simulink library "lib_lqr_controller"  (R2018a)
settings: Solver=VariableStepAuto  StartTime=0.0  StopTime=10.0  RelTol=1e-3
settings Model: Creator=aj  LastModifiedBy=aj

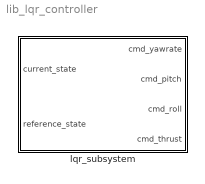
== system lib_lqr_controller ==
  lqr_subsystem : Subsystem  mask{lqr_k_matrix=[eye(3), eye(3), 0; zeros(1,6), 1], lqr_k_matrix_vel=[eye(3), eye(3), 0; zeros(1,6), 1], velcontrol_mode=off, total_mass_inair=0.85, gravity_accel=9.81}
      mask prompts: lqr_k_matrix "Feedback (fullstate) Gain Matrix [4x7]"; lqr_k_matrix_vel "Feedback (velocity) Gain Matrix [4x7]"; velcontrol_mode "Apply Only Velocity Control"; total_mass_inair "Total Flying Mass (kg)"; gravity_accel "Acceleration Due To Gravity"
      mask help:
      | This is the LQR control block.
      | Note: block color changes to 'lightBlue' if you are doing velocity-only control.
      mask Callback velcontrol_mode:
      | if( strcmp(get_param( gcb, 'velcontrol_mode' ), 'on') )
      |   set_param( gcb, 'BackgroundColor', 'lightBlue' );
      | else
      |   set_param( gcb, 'BackgroundColor', 'white' );
      | end
      mask DialogControl DescGroupVar Prompt: Nimbus LQR Block
      mask DialogControl DescTextVar Prompt: Generalized LQR feedback implemented as Simulink blocks.
      mask DialogControl Container3 Prompt: Specific Parameters

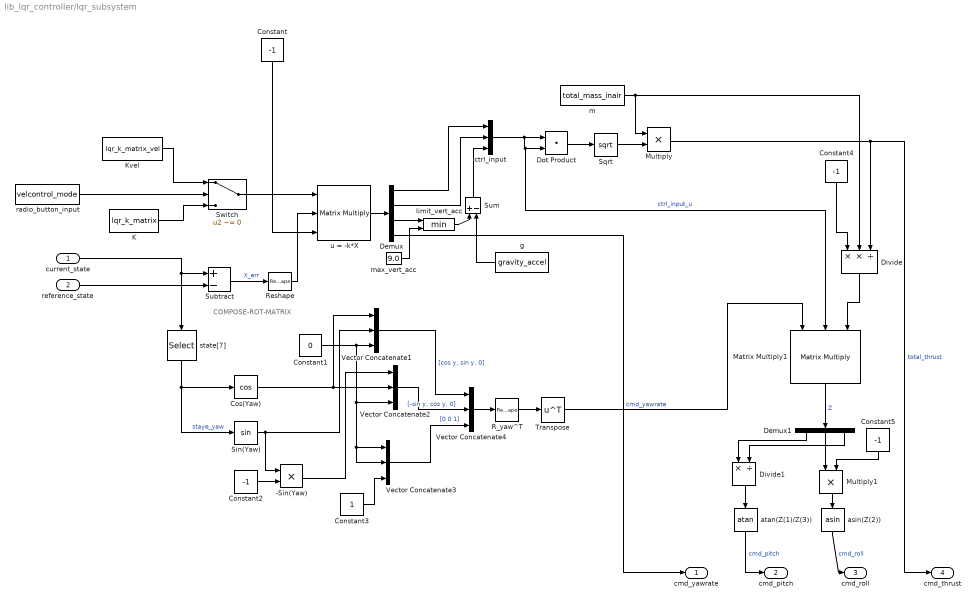
== system lib_lqr_controller/lqr_subsystem ==
  note: COMPOSE-ROT-MATRIX
  current_state : Inport  PortDimensions=7
  reference_state : Inport  Port=2
  -Sin(Yaw) : Product
  Constant{,2,4..5} (4 alike) : Constant  Value=-1
  Constant1 : Constant  Value=0
  Constant3 : Constant
  Cos(Yaw) : Trigonometry  Operator=cos
  Demux : Demux
  Demux1 : Demux  Outputs=3
  Divide : Product  Inputs=**/
  Divide1 : Product  Inputs=*/
  Dot Product : DotProduct  OutMin=0.001  InputSameDT=on  OutDataTypeStr=Inherit: Inherit via internal rule
  K : Constant  Value=lqr_k_matrix
  Kvel : Constant  Value=lqr_k_matrix_vel
  Matrix Multiply1 : Product  Inputs=3  Multiplication=Matrix(*)
  Multiply : Product
  Multiply1 : Product
  R_yaw^T : Reshape  OutputDimensionality=Customize  OutputDimensions=[3,3]
  Reshape : Reshape  OutputDimensionality=Column vector (2-D)
  Sin(Yaw) : Trigonometry
  Sqrt : Sqrt  SaturateOnIntegerOverflow=on
  Subtract : Sum  Inputs=+-
  Sum : Sum  Inputs=+-
  Switch : Switch  Criteria=u2 ~= 0
  Transpose : Math  Operator=transpose  SaturateOnIntegerOverflow=on
  Vector Concatenate{1..4} (4 alike) : Concatenate  NumInputs=3
  asin(Z(2)) : Trigonometry  Operator=asin
  atan(Z(1)/Z(3)) : Trigonometry  Operator=atan
  ctrl_input : Concatenate  NumInputs=3
  g : Constant  Value=gravity_accel
  limit_vert_acc : MinMax  Inputs=2
  m : Constant  Value=total_mass_inair
  max_vert_acc : Constant  Value=9.0
  radio_button_input : Constant  Value=velcontrol_mode
  state[7] : Selector  InputPortWidth=7  IndexOptions=Index vector (dialog)  Indices=7  OutputSizes=1
  u = -k*X : Product  Inputs=3  Multiplication=Matrix(*)
  cmd_yawrate : Outport
  cmd_pitch : Outport  Port=2
  cmd_roll : Outport  Port=3
  cmd_thrust : Outport  Port=4
  wires:
  R_yaw^T/1 -> Transpose/1
  Sqrt/1 -> Multiply/2
  u = -k*X/1 -> Demux/1
  g/1 -> Sum/2
  Demux1/3 -> Divide1/2
  Constant/1 -> u = -k*X/3
  Constant4/1 -> Divide/1
  Vector Concatenate3/1 -> Vector Concatenate4/3  "[0 0 1]"
  Demux1/1 -> Divide1/1
  Vector Concatenate2/1 -> Vector Concatenate4/2  "[-sin y, cos y, 0]"
  Constant2/1 -> -Sin(Yaw)/2
  Matrix Multiply1/1 -> Demux1/1  "Z"
  Vector Concatenate1/1 -> Vector Concatenate4/1  "[cos y, sin y, 0]"
  Transpose/1 -> Matrix Multiply1/1
  ctrl_input/1 -> Matrix Multiply1/2, Dot Product/2, Dot Product/1  "ctrl_input_u"
  Multiply/1 -> Divide/3, cmd_thrust/1  "total_thrust"
  Sin(Yaw)/1 -> Vector Concatenate1/2, -Sin(Yaw)/1
  m/1 -> Multiply/1, Divide/2
  Demux/3 -> limit_vert_acc/1
  Divide1/1 -> atan(Z(1)/Z(3))/1
  Demux/1 -> ctrl_input/1
  current_state/1 -> state[7]/1, Subtract/1
  atan(Z(1)/Z(3))/1 -> cmd_pitch/1  "cmd_pitch"
  Demux/2 -> ctrl_input/2
  Divide/1 -> Matrix Multiply1/3
  Demux1/2 -> Multiply1/1
  Constant3/1 -> Vector Concatenate3/3
  Cos(Yaw)/1 -> Vector Concatenate2/2, Vector Concatenate1/1
  Demux/4 -> cmd_yawrate/1  "cmd_yawrate"
  -Sin(Yaw)/1 -> Vector Concatenate2/1
  Sum/1 -> ctrl_input/3
  Vector Concatenate4/1 -> R_yaw^T/1
  Dot Product/1 -> Sqrt/1
  Constant1/1 -> Vector Concatenate3/1, Vector Concatenate3/2, Vector Concatenate2/3, Vector Concatenate1/3
  state[7]/1 -> Sin(Yaw)/1, Cos(Yaw)/1  "staye_yaw"
  reference_state/1 -> Subtract/2
  asin(Z(2))/1 -> cmd_roll/1  "cmd_roll"
  Subtract/1 -> Reshape/1  "X_err"
  Reshape/1 -> u = -k*X/2
  K/1 -> Switch/3
  Constant5/1 -> Multiply1/2
  Multiply1/1 -> asin(Z(2))/1
  Kvel/1 -> Switch/1
  radio_button_input/1 -> Switch/2
  Switch/1 -> u = -k*X/1
  max_vert_acc/1 -> limit_vert_acc/2
  limit_vert_acc/1 -> Sum/1
